simulink model "prius_nocontrol"  (Simulink 6.0)
settings: Solver=ode4  SolverMode=SingleTasking  StartTime=0.0  StopTime=time_final  FixedStep=time_step  RelTol=1e-3  AbsTol=1e-6
values from neighbouring files (symbols this model uses):
  A_frontal = 2.52    [prius_sim_data.m]
  C_d = 0.3    [prius_sim_data.m]
  enable_stop = 1    [prius_sim_data.m]
  eng_consum_fuel = [0 0.654 0.328 0.238 0.232 0.257 0.29 0.323 0.353 0.381 0.407 0.435 0.465 0.501 0.545 0.599 0.665 0.746 0.842 0.957 ... (first row only)    [prius_sim_data.m]
  ess_cap_scale = 1    [prius_sim_data.m]
  ess_fixtemp = 40    [prius_sim_data.m]
  ess_init_soc = soc_init_index(simrun)    [prius_sim_init.m]
  ess_max_ah_cap = [6.0 6.0]    [prius_sim_data.m]
  ess_max_volts = 9    [prius_sim_data.m]
  ess_min_volts = 6    [prius_sim_data.m]
  ess_module_num = 40    [prius_sim_data.m]
  ess_res_scale_coef = [1 0 1 0]    [prius_sim_data.m]
  ess_res_scale_fun = inline('(x(1)*ess_module_num+x(2))/(x(3)*ess_cap_scale+x(4))','x','ess_module_num','ess_cap_scale')    [prius_sim_data.m]
  ess_tmp = [0 25]    [prius_sim_data.m]
  f_rolling = 0.015    [prius_sim_data.m]
  FR = 3.905    [prius_sim_data.m]
  g_eff_map = 0.95*[ 0.88	0.89	0.90	0.91	0.90	0.79	0.79	0.79	0.90	0.91	0.90	0.89	0.88 ... (first row only)    [prius_sim_data.m]
  g_gravity = 9.81    [prius_sim_data.m]
  g_max_spd = [-200000 -10000 -8000 -6500 -5500 -4000 -3500 -3000 -2500 -2000 -1500 -1000 -500 0 500 1000 1500 2000 2500 3000 3500 4000 5500 6500 8000 10000 200000]*(2*pi)/60    [prius_sim_data.m]
  g_max_trq = 1.2*[0.01 14.3 18 22 26 36 41 48 55 55 55 55 55 55 55 55 55 55 55 48 41 36 26 22 18 14.3 0.01]    [prius_sim_data.m]
  gear_no = 4    [prius_sim_data.m]
  m_eff_map = 0.95*[ .905    .905    .905    .905    .905    .905    .905    .905    .905    .905    .905    .905	.905    .905    .905    .905    .905    .905    .905    .905    .905    .905    .905 ... (first row only)    [prius_sim_data.m]
  m_map_spd = [0 500 1000 1500 2000 2500 3000 3500 4000 4500  6000]*(2*pi)/60    [prius_sim_data.m]
  m_max_trq = interp1(m_spd_data,m_max_trq_data,m_map_spd,'linear')    [prius_sim_data.m]
  m_min_volts = 60    [prius_sim_data.m]
  M_total = 1.254*10^3    (= 1254)    [prius_sim_data.m]
  R_tire = 0.287    [prius_sim_data.m]
  rho_air = 1.2    [prius_sim_data.m]
  T2W = inv(W2T)    [prius_sim_data.m]
  time_final = 1*length(cyc_mph(:,2))    [prius_sim_init.m]
  tx_pg_r = 78    [prius_sim_data.m]
  tx_pg_s = 30    [prius_sim_data.m]
undefined symbols (not defined in the file or in its folder): eng_map_trq
settings Model: LastModifiedBy=cpdguest  ExtModeTrigMode=oneshot  ExtModeArmWhenConnect=off  BufferReuse=off
settings SolverCC: InitialStep=0.001
settings DataIOCC: LimitDataPoints=off  SaveOutput=off  SaveTime=off  SignalLoggingName=sigsOut
settings OptimizationCC: BooleanDataType=off  InlineInvariantSignals=off  OptimizeBlockIOStorage=off  BufferReuse=off  ExpressionFolding=off  LocalBlockOutputs=off
settings DebuggingCC: SolverPrmCheckMsg=none
settings HardwareCC: TargetUnknown=on

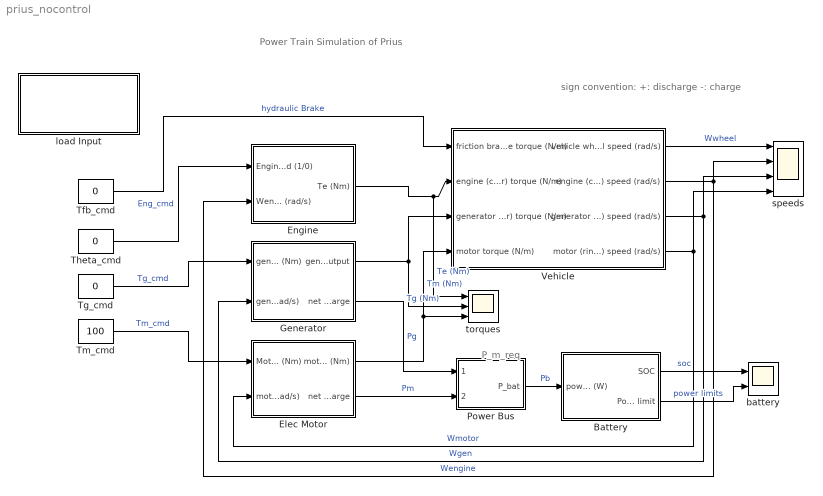
== system prius_nocontrol ==
  note: Power Train Simulation of Prius
  note: P_m_req
  note: sign convention:
      | +: discharge     -: charge
  Battery : Subsystem
      mask Display: disp('Battery')
  Elec Motor : Subsystem
      mask Display: disp('Electric\nMotor')
  Engine : Subsystem
      mask Display: disp('Engine')
  Generator : Subsystem
      mask Display: disp('Generator')
  Power Bus : Subsystem
      mask Display: disp('Power\nBus')
  Tfb_cmd : Constant  Value=0
  Tg_cmd : Constant  Value=0
  Theta_cmd : Constant  Value=0
  Tm_cmd : Constant  Value=100
  Vehicle : Subsystem
      mask Display: disp('Planetary Gear Set\n&\nVehicle')
  battery : Scope  NumInputPorts=2
      settings: TickLabels=on  TimeRange=30  YMin=0~-100  YMax=100~150  SaveName=ScopeData3
  load Input : Subsystem
      settings: OpenFcn=prius_sim_init
      mask Help: This block runs/ndes_init.m file in the main directory
      mask Display: disp('Load Input Data')
  speeds : Scope  NumInputPorts=4
      settings: TickLabels=on  TimeRange=30  YMin=0~-100~-100~-5  YMax=100~150~400~5
  torques : Scope  NumInputPorts=3
      settings: TickLabels=on  TimeRange=30  YMin=0~-100~-100  YMax=100~150~400  SaveName=ScopeData7
  wires:
  Power Bus/1(P_bat) -> Battery/1(power req'd into bus (W))  "Pb"
  Theta_cmd/1 -> Engine/1(Engine on/off cmd (1/0))  "Eng_cmd"
  Tg_cmd/1 -> Generator/1(generator command Torque (Nm))  "Tg_cmd"
  Tm_cmd/1 -> Elec Motor/1(Motor demand Torque (Nm))  "Tm_cmd"
  Elec Motor/2(net Power >0 discharge  <0 charge) -> Power Bus/2(P_motor)  "Pm"
  Generator/2(net Power <0 discharge  >0 charge) -> Power Bus/1(P_generator)  "Pg"
  Tfb_cmd/1 -> Vehicle/1(friction brake torque (N/m))  "hydraulic Brake"
  Engine/1(Te (Nm)) -> Vehicle/2(engine (carrier) torque (N/m)), torques/1  "Te (Nm)"
  Vehicle/2(engine (carrier) speed (rad/s)) -> Engine/2(Wengine (rad/s)), speeds/2  "Wengine"
  Vehicle/3(generator (sun gear) speed (rad/s)) -> Generator/2(generator speed (rad/s)), speeds/3  "Wgen"
  Vehicle/4(motor (ring gear) speed (rad/s)) -> Elec Motor/2(motor speed (rad/s)), speeds/4  "Wmotor"
  Generator/1(generator torque output) -> Vehicle/3(generator (sun gear) torque (N/m)), torques/2  "Tg (Nm)"
  Elec Motor/1(motor torque output (Nm)) -> Vehicle/4(motor torque (N/m)), torques/3  "Tm (Nm)"
  Vehicle/1(vehicle wheel speed (rad/s)) -> speeds/1  "Wwheel"
  Battery/1(SOC) -> battery/1  "soc"
  Battery/2(Power limit) -> battery/2  "power limits"

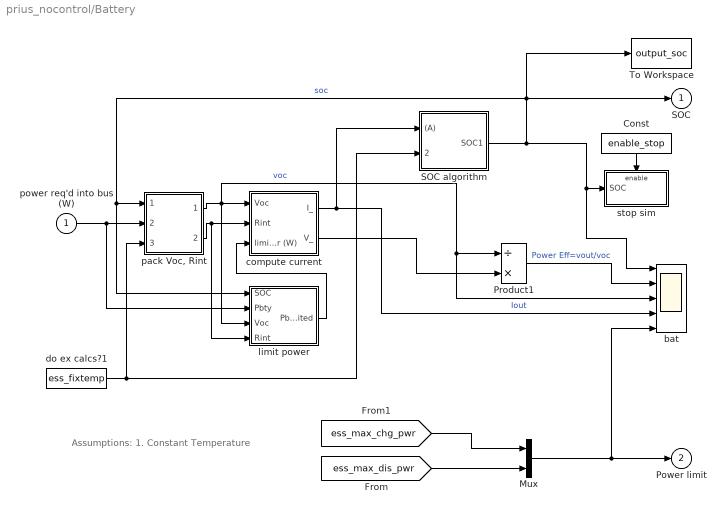
== system prius_nocontrol/Battery ==
  note: Assumptions:
      | 1. Constant Temperature
  power req'd into bus (W) : Inport  Port=1  LatchInput=off
  Const : Constant  Orientation=down  Value=enable_stop
  Mux : Mux  Inputs=2
  Product1 : Product  Inputs=/*  SaturateOnIntegerOverflow=on  InputSameDT=on
  SOC algorithm : Subsystem  AncestorBlock=|
      | lib_energy_storage/Ess Choices/energy
      | storage <ess>/SOC
      | algorithm
      mask Display: disp('SOC\nalgorithm')
  To Workspace : ToWorkspace  VariableName=output_soc  SampleTime=-1  SaveFormat=Array
  bat : Scope  NumInputPorts=5
      settings: TimeRange=367  YMin=0.25~0.75~302~-75~-30000  YMax=0.65~1.2~310~75~25000
  compute current : Subsystem  AncestorBlock=|
      | lib_energy_storage/Ess Choices/energy
      | storage <ess>/compute
      | current
      mask Display: disp('Compute\nCurrent')
  do ex calcs?1 : Constant  Value=ess_fixtemp
  limit power : Subsystem  AncestorBlock=lib_energy_storage/Ess Choices/energy storage <ess>/limit power
      mask Display: disp('Limit\nPower')
  "pack Voc, Rint" : Subsystem  AncestorBlock=|
      | lib_energy_storage/Ess Choices/energy
      | storage <ess>/pack
      | Voc, Rint
      mask Display: disp('Pack\nVoc,Rint')
  stop sim : Subsystem  AncestorBlock=lib_energy_storage/Ess Choices/energy storage <ess>/stop sim  TreatAsAtomicUnit=on
  SOC : Outport  InitialOutput=0
  Power limit : Outport  Port=2  InitialOutput=0
  wires:
  limit power/1("Pbty, limited") -> compute current/3(limited output power (W))
  "pack Voc, Rint"/1(pack open- circuit voltage) -> limit power/3(Voc), compute current/1(Voc), Product1/1, bat/3  "voc"
  "pack Voc, Rint"/2(pack resistance) -> compute current/2(Rint), limit power/4(Rint)
  Const/1 -> stop sim/Enable
  SOC algorithm/1(SOC1) -> limit power/1(SOC), "pack Voc, Rint"/1(SOC (prev)), SOC/1, To Workspace/1, bat/1, stop sim/1(SOC)  "soc"
  compute current/1(I_) -> SOC algorithm/1((A)), bat/4  "Iout"
  power req'd into bus (W)/1 -> "pack Voc, Rint"/2(req'd battery power (W)), limit power/2(Pbty)
  compute current/2(V_) -> Product1/2
  do ex calcs?1/1 -> "pack Voc, Rint"/3(mod tmp   (C)), SOC algorithm/2(tmp (C))
  Mux/1 -> Power limit/1, bat/5
  Product1/1 -> bat/2  "Power Eff=vout/voc"
  [ess_max_dis_pwr] -> Mux/2
  [ess_max_chg_pwr] -> Mux/1

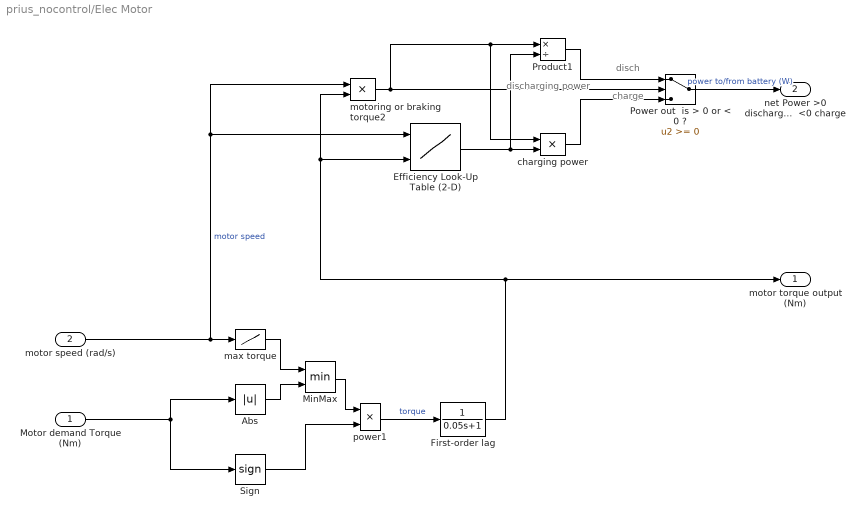
== system prius_nocontrol/Elec Motor ==
  note: disch
  note: charge
  note: discharging
      | power
  Motor demand Torque (Nm) : Inport  Port=1  LatchInput=off
  motor speed (rad/s) : Inport  Port=2  LatchInput=off
  Abs : Abs  SaturateOnIntegerOverflow=on
  Efficiency Look-Up Table (2-D) : Lookup2D  DialogController=Simulink.DDGSource  RowIndex=m_map_spd  ColumnIndex=m_map_trq  OutputValues=m_eff_map  SaturateOnIntegerOverflow=on  InputSameDT=on
  First-order lag : TransferFcn  Denominator=[0.05 1]
  MinMax : MinMax  Inputs=2  SaturateOnIntegerOverflow=on  InputSameDT=on
  Power out  is > 0 or < 0 ? : Switch  SaturateOnIntegerOverflow=on  InputSameDT=on
  Product1 : Product  Inputs=*/  SaturateOnIntegerOverflow=on  InputSameDT=on
  Sign : Signum
  charging power : Product  SaturateOnIntegerOverflow=on  InputSameDT=on
  max torque : Lookup  DialogController=Simulink.DDGSource  InputValues=m_map_spd  OutputValues=m_max_trq  SaturateOnIntegerOverflow=on
  motoring or braking torque2 : Product  SaturateOnIntegerOverflow=on  InputSameDT=on
  power1 : Product  SaturateOnIntegerOverflow=on  InputSameDT=on
  motor torque output (Nm) : Outport  InitialOutput=0
  net Power >0 discharge  <0 charge : Outport  Port=2  InitialOutput=0
  wires:
  charging power/1 -> Power out  is > 0 or < 0 ?/3
  Product1/1 -> Power out  is > 0 or < 0 ?/1
  Power out  is > 0 or < 0 ?/1 -> net Power >0 discharge  <0 charge/1  "power to/from battery (W)"
  motor speed (rad/s)/1 -> Efficiency Look-Up Table (2-D)/1, motoring or braking torque2/1, max torque/1  "motor speed"
  Motor demand Torque (Nm)/1 -> Abs/1, Sign/1
  power1/1 -> First-order lag/1  "torque"
  Efficiency Look-Up Table (2-D)/1 -> Product1/2, charging power/2
  motoring or braking torque2/1 -> Product1/1, charging power/1, Power out  is > 0 or < 0 ?/2
  Abs/1 -> MinMax/2
  max torque/1 -> MinMax/1
  MinMax/1 -> power1/1
  Sign/1 -> power1/2
  First-order lag/1 -> Efficiency Look-Up Table (2-D)/2, motoring or braking torque2/2, motor torque output (Nm)/1

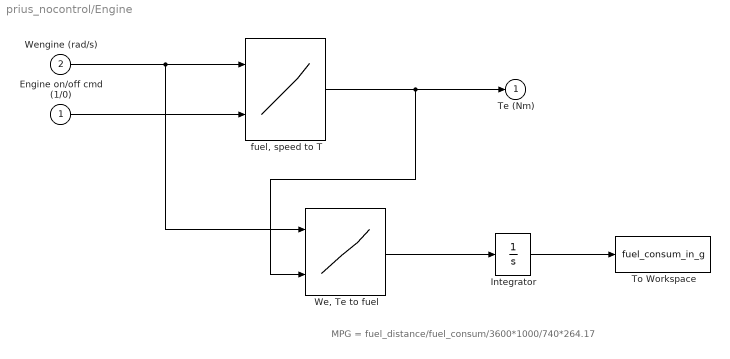
== system prius_nocontrol/Engine ==
  note: MPG = fuel_distance/fuel_consum/3600*1000/740*264.17
  Engine on/off cmd (1/0) : Inport  Port=1  LatchInput=off
  Wengine (rad/s) : Inport  Port=2  LatchInput=off
  Integrator : Integrator  UpperSaturationLimit=20.5  LowerSaturationLimit=0
  To Workspace : ToWorkspace  VariableName=fuel_consum_in_g  SampleTime=time_final  SaveFormat=Array
  "We, Te to fuel" : Lookup2D  DialogController=Simulink.DDGSource  RowIndex=eng_consum_spd  ColumnIndex=eng_consum_trq  OutputValues=eng_consum_fuel  SaturateOnIntegerOverflow=on  InputSameDT=on
  "fuel, speed to T" : Lookup2D  DialogController=Simulink.DDGSource  RowIndex=eng_map_spd  ColumnIndex=eng_map_fuel  OutputValues=eng_map_trq  SaturateOnIntegerOverflow=on  InputSameDT=on
  Te (Nm) : Outport
  wires:
  Engine on/off cmd (1/0)/1 -> "fuel, speed to T"/2
  Wengine (rad/s)/1 -> "fuel, speed to T"/1, "We, Te to fuel"/1
  "fuel, speed to T"/1 -> Te (Nm)/1, "We, Te to fuel"/2
  "We, Te to fuel"/1 -> Integrator/1
  Integrator/1 -> To Workspace/1

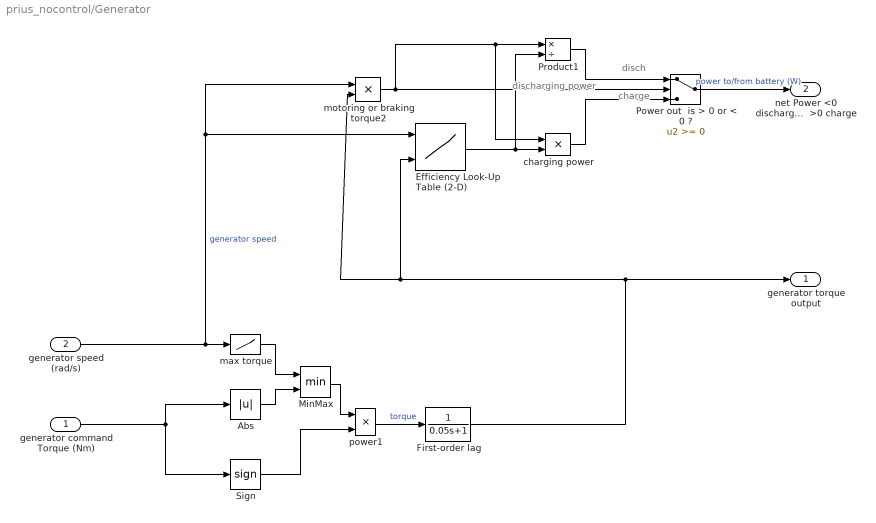
== system prius_nocontrol/Generator ==
  note: disch
  note: charge
  note: discharging
      | power
  generator command Torque (Nm) : Inport  Port=1  LatchInput=off
  generator speed (rad/s) : Inport  Port=2  LatchInput=off
  Abs : Abs  SaturateOnIntegerOverflow=on
  Efficiency Look-Up Table (2-D) : Lookup2D  DialogController=Simulink.DDGSource  RowIndex=g_map_spd  ColumnIndex=g_map_trq  OutputValues=g_eff_map  SaturateOnIntegerOverflow=on  InputSameDT=on
  First-order lag : TransferFcn  Denominator=[0.05 1]
  MinMax : MinMax  Inputs=2  SaturateOnIntegerOverflow=on  InputSameDT=on
  Power out  is > 0 or < 0 ? : Switch  SaturateOnIntegerOverflow=on  InputSameDT=on
  Product1 : Product  Inputs=*/  SaturateOnIntegerOverflow=on  InputSameDT=on
  Sign : Signum
  charging power : Product  SaturateOnIntegerOverflow=on  InputSameDT=on
  max torque : Lookup  DialogController=Simulink.DDGSource  InputValues=g_max_spd  OutputValues=g_max_trq  SaturateOnIntegerOverflow=on
  motoring or braking torque2 : Product  SaturateOnIntegerOverflow=on  InputSameDT=on
  power1 : Product  SaturateOnIntegerOverflow=on  InputSameDT=on
  generator torque output : Outport  InitialOutput=0
  net Power <0 discharge  >0 charge : Outport  Port=2  InitialOutput=0
  wires:
  charging power/1 -> Power out  is > 0 or < 0 ?/3
  Product1/1 -> Power out  is > 0 or < 0 ?/1
  Power out  is > 0 or < 0 ?/1 -> net Power <0 discharge  >0 charge/1  "power to/from battery (W)"
  generator speed (rad/s)/1 -> Efficiency Look-Up Table (2-D)/1, motoring or braking torque2/1, max torque/1  "generator speed"
  generator command Torque (Nm)/1 -> Abs/1, Sign/1
  power1/1 -> First-order lag/1  "torque"
  Efficiency Look-Up Table (2-D)/1 -> Product1/2, charging power/2
  motoring or braking torque2/1 -> Product1/1, charging power/1, Power out  is > 0 or < 0 ?/2
  Abs/1 -> MinMax/2
  max torque/1 -> MinMax/1
  MinMax/1 -> power1/1
  Sign/1 -> power1/2
  First-order lag/1 -> generator torque output/1, Efficiency Look-Up Table (2-D)/2, motoring or braking torque2/2

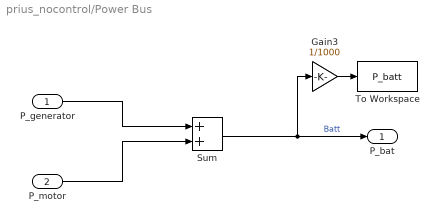
== system prius_nocontrol/Power Bus ==
  P_generator : Inport  Port=1  LatchInput=off
  P_motor : Inport  Port=2  LatchInput=off
  Gain3 : Gain  Gain=1/1000  SaturateOnIntegerOverflow=on
  Sum : Sum  SaturateOnIntegerOverflow=on  InputSameDT=on
  To Workspace : ToWorkspace  VariableName=P_batt  SampleTime=-1  SaveFormat=Array
  P_bat : Outport  InitialOutput=0
  wires:
  P_generator/1 -> Sum/1
  P_motor/1 -> Sum/2
  Sum/1 -> P_bat/1, Gain3/1  "Batt"
  Gain3/1 -> To Workspace/1

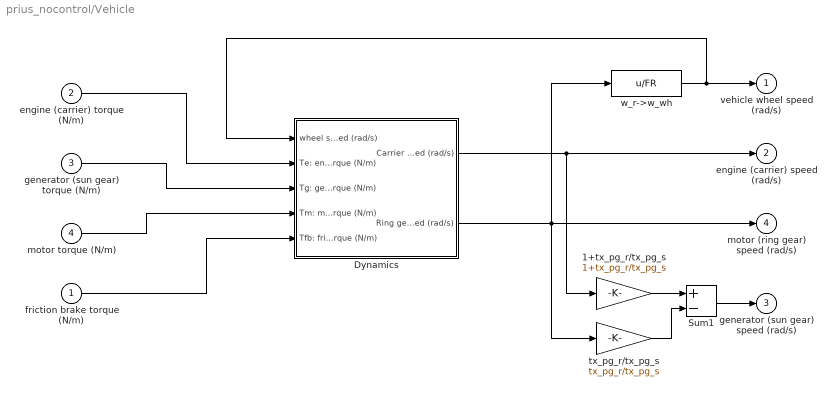
== system prius_nocontrol/Vehicle ==
  friction brake torque (N/m) : Inport  Port=1  LatchInput=off
  engine (carrier) torque (N/m) : Inport  Port=2  LatchInput=off
  generator (sun gear) torque (N/m) : Inport  Port=3  LatchInput=off
  motor torque (N/m) : Inport  Port=4  LatchInput=off
  1+tx_pg_r/tx_pg_s : Gain  Gain=1+tx_pg_r/tx_pg_s  SaturateOnIntegerOverflow=on
  Dynamics : Subsystem
      mask Display: disp('Dynamic Model\nTwo DOF')
  Sum1 : Sum  Inputs=+-  SaturateOnIntegerOverflow=on  InputSameDT=on
  tx_pg_r/tx_pg_s : Gain  Gain=tx_pg_r/tx_pg_s  SaturateOnIntegerOverflow=on
  w_r->w_wh : Fcn  Expr=u/FR
  vehicle wheel speed (rad/s) : Outport
  engine (carrier) speed (rad/s) : Outport  Port=2
  generator (sun gear) speed (rad/s) : Outport  Port=3
  motor (ring gear) speed (rad/s) : Outport  Port=4
  wires:
  tx_pg_r/tx_pg_s/1 -> Sum1/2
  1+tx_pg_r/tx_pg_s/1 -> Sum1/1
  engine (carrier) torque (N/m)/1 -> Dynamics/2(Te: engine (carrier) torque (N/m))
  motor torque (N/m)/1 -> Dynamics/4(Tm: motor torque (N/m))
  friction brake torque (N/m)/1 -> Dynamics/5("Tfb: friction brake torque (N/m) ")
  w_r->w_wh/1 -> vehicle wheel speed (rad/s)/1, Dynamics/1(wheel speed (rad/s))
  generator (sun gear) torque (N/m)/1 -> Dynamics/3(Tg: generator (sun gear) torque (N/m))
  Sum1/1 -> generator (sun gear) speed (rad/s)/1
  Dynamics/1(Carrier speed (rad/s)) -> engine (carrier) speed (rad/s)/1, 1+tx_pg_r/tx_pg_s/1
  Dynamics/2(Ring gear speed (rad/s)) -> w_r->w_wh/1, motor (ring gear) speed (rad/s)/1, tx_pg_r/tx_pg_s/1

== system prius_nocontrol/load Input ==
  note: double_click to load

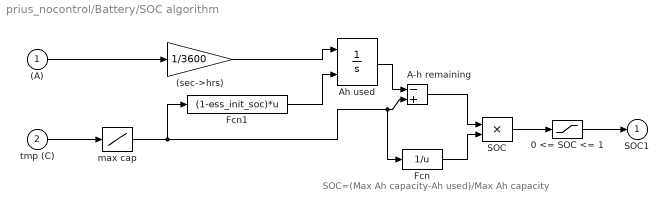
== system prius_nocontrol/Battery/SOC algorithm ==
  note: SOC=(Max Ah capacity-Ah used)/Max Ah capacity
  (A) : Inport  Port=1  LatchInput=off
  tmp (C) : Inport  Port=2  LatchInput=off
  (sec->hrs) : Gain  Gain=1/3600  SaturateOnIntegerOverflow=on
  0 <= SOC <= 1 : Saturate  UpperLimit=1  LowerLimit=0
  A-h remaining : Sum  Inputs=-+  SaturateOnIntegerOverflow=on  InputSameDT=on
  Ah used : Integrator  InitialConditionSource=external  InitialCondition=(1-ess_init_soc)*ess_max_ah_cap
  Fcn : Fcn  Expr=1/u
  Fcn1 : Fcn  Expr=(1-ess_init_soc)*u
  SOC : Product  SaturateOnIntegerOverflow=on  InputSameDT=on
  max cap : Lookup  DialogController=Simulink.DDGSource  InputValues=ess_tmp  OutputValues=ess_max_ah_cap*ess_cap_scale  SaturateOnIntegerOverflow=on
  SOC1 : Outport  InitialOutput=0
  wires:
  (A)/1 -> (sec->hrs)/1
  (sec->hrs)/1 -> Ah used/1
  Ah used/1 -> A-h remaining/1
  Fcn/1 -> SOC/2
  SOC/1 -> 0 <= SOC <= 1/1
  A-h remaining/1 -> SOC/1
  0 <= SOC <= 1/1 -> SOC1/1
  tmp (C)/1 -> max cap/1
  max cap/1 -> A-h remaining/2, Fcn/1, Fcn1/1
  Fcn1/1 -> Ah used/2

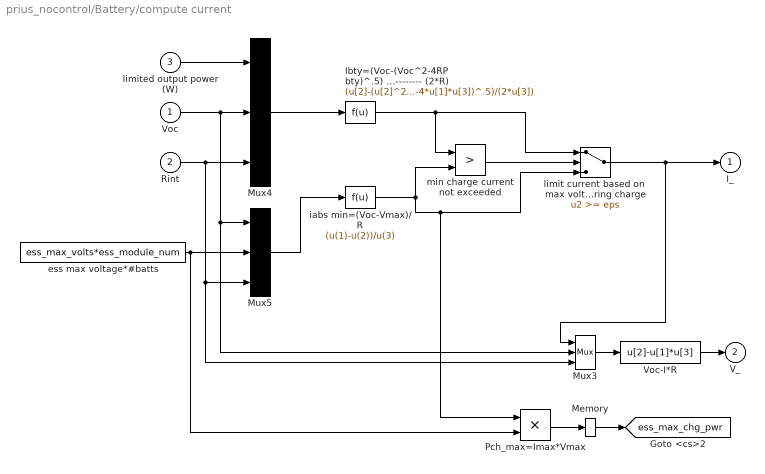
== system prius_nocontrol/Battery/compute current ==
  Voc : Inport  Port=1  LatchInput=off
  Rint : Inport  Port=2  LatchInput=off
  limited output power (W) : Inport  Port=3  LatchInput=off
  Ibty=(Voc-(Voc^2-4RPbty)^.5)        ----------------------------- (2*R) : Fcn  Expr=(u[2]-(u[2]^2-4*u[1]*u[3])^.5)/(2*u[3])
  Memory : Memory
  Mux3 : Mux  Inputs=3
  Mux4 : Mux  Inputs=3
  Mux5 : Mux  Inputs=3
  Pch_max=Imax*Vmax : Product  SaturateOnIntegerOverflow=on  InputSameDT=on
  Voc-I*R : Fcn  Expr=u[2]-u[1]*u[3]
  ess max voltage*#batts : Constant  Value=ess_max_volts*ess_module_num
  iabs min=(Voc-Vmax)/R : Fcn  Expr=(u(1)-u(2))/u(3)
  limit current based on  max voltage during charge : Switch  Threshold=eps  SaturateOnIntegerOverflow=on  InputSameDT=on
  min charge current not exceeded : RelationalOperator  Operator=>  InputSameDT=on
  I_ : Outport  InitialOutput=0
  V_ : Outport  Port=2  InitialOutput=0
  tag scope: ess_max_chg_pwr=global
  wires:
  limited output power (W)/1 -> Mux4/1
  Voc/1 -> Mux4/2, Mux3/2, Mux5/1
  Rint/1 -> Mux4/3, Mux3/3, Mux5/3
  Ibty=(Voc-(Voc^2-4RPbty)^.5)        ----------------------------- (2*R)/1 -> min charge current not exceeded/1, limit current based on  max voltage during charge/1
  iabs min=(Voc-Vmax)/R/1 -> min charge current not exceeded/2, limit current based on  max voltage during charge/3, Pch_max=Imax*Vmax/1
  limit current based on  max voltage during charge/1 -> Mux3/1, I_/1
  min charge current not exceeded/1 -> limit current based on  max voltage during charge/2
  Mux3/1 -> Voc-I*R/1
  Voc-I*R/1 -> V_/1
  Mux4/1 -> Ibty=(Voc-(Voc^2-4RPbty)^.5)        ----------------------------- (2*R)/1
  Mux5/1 -> iabs min=(Voc-Vmax)/R/1
  ess max voltage*#batts/1 -> Mux5/2, Pch_max=Imax*Vmax/2
  Pch_max=Imax*Vmax/1 -> Memory/1
  Memory/1 -> [ess_max_chg_pwr]

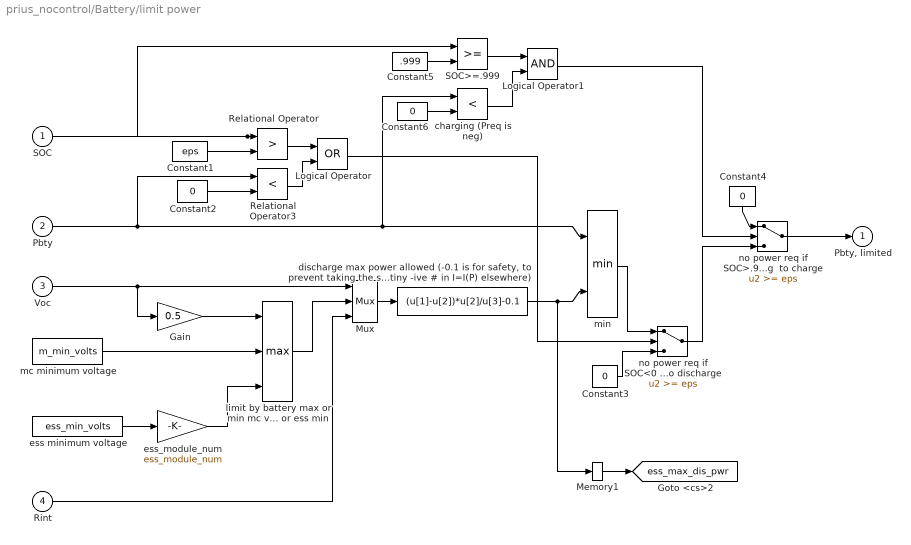
== system prius_nocontrol/Battery/limit power ==
  SOC : Inport  Port=1  LatchInput=off
  Pbty : Inport  Port=2  LatchInput=off
  Voc : Inport  Port=3  LatchInput=off
  Rint : Inport  Port=4  LatchInput=off
  Constant1 : Constant  Value=eps
  Constant2 : Constant  Value=0
  Constant3 : Constant  Value=0
  Constant4 : Constant  Orientation=down  Value=0
  Constant5 : Constant  Value=.999
  Constant6 : Constant  Value=0
  Gain : Gain  Gain=0.5  SaturateOnIntegerOverflow=on
  Logical Operator : Logic  Operator=OR
  Logical Operator1 : Logic
  Memory1 : Memory
  Mux : Mux  Inputs=3
  Relational Operator : RelationalOperator  Operator=>  InputSameDT=on
  Relational Operator3 : RelationalOperator  Operator=<  InputSameDT=on
  SOC>=.999 : RelationalOperator  InputSameDT=on
  charging (Preq is neg) : RelationalOperator  Operator=<  InputSameDT=on
  "discharge max power allowed (-0.1 is for safety, to prevent taking the square of a tiny -ive # in I=I(P) elsewhere)" : Fcn  Expr=(u[1]-u[2])*u[2]/u[3]-0.1
  ess minimum voltage : Constant  Value=ess_min_volts
  ess_module_num : Gain  Gain=ess_module_num  SaturateOnIntegerOverflow=on
  limit by battery max or min mc voltage or ess min : MinMax  Function=max  Inputs=3  SaturateOnIntegerOverflow=on  InputSameDT=on
  mc minimum voltage : Constant  Value=m_min_volts
  min : MinMax  Inputs=2  SaturateOnIntegerOverflow=on  InputSameDT=on
  no power req if SOC<0 and trying  to discharge : Switch  Threshold=eps  SaturateOnIntegerOverflow=on  InputSameDT=on
  no power req if SOC>.999 and trying  to charge : Switch  Threshold=eps  SaturateOnIntegerOverflow=on  InputSameDT=on
  "Pbty, limited" : Outport  InitialOutput=0
  tag scope: ess_max_dis_pwr=global
  wires:
  Constant1/1 -> Relational Operator/2
  Relational Operator/1 -> Logical Operator/1
  Pbty/1 -> Relational Operator3/1, charging (Preq is neg)/1, min/1
  Constant2/1 -> Relational Operator3/2
  Relational Operator3/1 -> Logical Operator/2
  Constant3/1 -> no power req if SOC<0 and trying  to discharge/3
  Logical Operator/1 -> no power req if SOC<0 and trying  to discharge/2
  Voc/1 -> Mux/1, Gain/1
  min/1 -> no power req if SOC<0 and trying  to discharge/1
  Mux/1 -> "discharge max power allowed (-0.1 is for safety, to prevent taking the square of a tiny -ive # in I=I(P) elsewhere)"/1
  limit by battery max or min mc voltage or ess min/1 -> Mux/2
  "discharge max power allowed (-0.1 is for safety, to prevent taking the square of a tiny -ive # in I=I(P) elsewhere)"/1 -> min/2, Memory1/1
  mc minimum voltage/1 -> limit by battery max or min mc voltage or ess min/2
  Rint/1 -> Mux/3
  Gain/1 -> limit by battery max or min mc voltage or ess min/1
  ess minimum voltage/1 -> ess_module_num/1
  ess_module_num/1 -> limit by battery max or min mc voltage or ess min/3
  SOC/1 -> Relational Operator/1, SOC>=.999/1
  SOC>=.999/1 -> Logical Operator1/1
  Constant6/1 -> charging (Preq is neg)/2
  charging (Preq is neg)/1 -> Logical Operator1/2
  Constant5/1 -> SOC>=.999/2
  Constant4/1 -> no power req if SOC>.999 and trying  to charge/1
  no power req if SOC<0 and trying  to discharge/1 -> no power req if SOC>.999 and trying  to charge/3
  no power req if SOC>.999 and trying  to charge/1 -> "Pbty, limited"/1
  Logical Operator1/1 -> no power req if SOC>.999 and trying  to charge/2
  Memory1/1 -> [ess_max_dis_pwr]

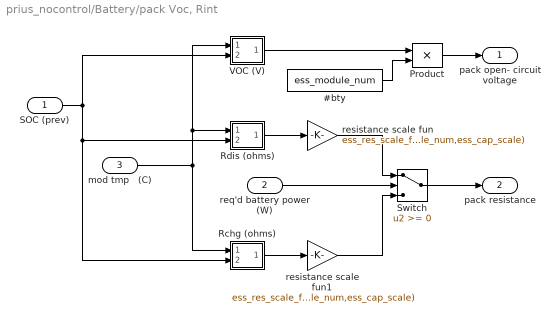
== system prius_nocontrol/Battery/pack Voc, Rint ==
  SOC (prev) : Inport  Port=1  LatchInput=off
  req'd battery power (W) : Inport  Port=2  LatchInput=off
  mod tmp   (C) : Inport  Port=3  LatchInput=off
  #bty : Constant  Value=ess_module_num
  Product : Product  SaturateOnIntegerOverflow=on  InputSameDT=on
  Rchg (ohms) : Subsystem  mask(2-D Table Lookup){@1=ess_tmp, @2=ess_soc, @3=ess_r_chg}
      mask prompts: @1 "X Index"; @2 "Y Index"; @3 "Table"
      mask help:
      | Two Dimensional Table Lookup
      | The first input corresponds to X Index and the second input corresponds to the Y Index
      mask init:
      | xindex=@1; yindex=@2; table=@3; sftab2chk(xindex,yindex,table);
      mask Help: This block returns a linearly interpolated intersection from the table using the X index (which corresponds to the rows of the table) and the Y index (which corresponds to the columns of the table).  Extrapolation is used.
      mask Display: plot(-10,-10,110,110,[90,50,10],[90,40,30],[90,50,10],[50,26,20],[90,50,10],[22,13,10])
  Rdis (ohms) : Subsystem  mask(2-D Table Lookup){@1=ess_tmp, @2=ess_soc, @3=ess_r_dis}
      mask prompts: @1 "X Index"; @2 "Y Index"; @3 "Table"
      mask help:
      | Two Dimensional Table Lookup
      | The first input corresponds to X Index and the second input corresponds to the Y Index
      mask init:
      | xindex=@1; yindex=@2; table=@3; sftab2chk(xindex,yindex,table);
      mask Help: This block returns a linearly interpolated intersection from the table using the X index (which corresponds to the rows of the table) and the Y index (which corresponds to the columns of the table).  Extrapolation is used.
      mask Display: plot(-10,-10,110,110,[90,50,10],[90,40,30],[90,50,10],[50,26,20],[90,50,10],[22,13,10])
  Switch : Switch  SaturateOnIntegerOverflow=on  InputSameDT=on
  VOC (V) : Subsystem  mask(2-D Table Lookup){@1=ess_tmp, @2=ess_soc, @3=ess_voc}
      mask prompts: @1 "X Index"; @2 "Y Index"; @3 "Table"
      mask help:
      | Two Dimensional Table Lookup
      | The first input corresponds to X Index and the second input corresponds to the Y Index
      mask init:
      | xindex=@1; yindex=@2; table=@3; sftab2chk(xindex,yindex,table);
      mask Help: This block returns a linearly interpolated intersection from the table using the X index (which corresponds to the rows of the table) and the Y index (which corresponds to the columns of the table).  Extrapolation is used.
      mask Display: plot(-10,-10,110,110,[90,50,10],[90,40,30],[90,50,10],[50,26,20],[90,50,10],[22,13,10])
  resistance scale fun : Gain  Gain=ess_res_scale_fun(ess_res_scale_coef,ess_module_num,ess_cap_scale)  SaturateOnIntegerOverflow=on
  resistance scale fun1 : Gain  Gain=ess_res_scale_fun(ess_res_scale_coef,ess_module_num,ess_cap_scale)  SaturateOnIntegerOverflow=on
  pack open- circuit voltage : Outport  InitialOutput=0
  pack resistance : Outport  Port=2  InitialOutput=0
  wires:
  resistance scale fun1/1 -> Switch/3
  Rchg (ohms)/1(table out) -> resistance scale fun1/1
  resistance scale fun/1 -> Switch/1
  Rdis (ohms)/1(table out) -> resistance scale fun/1
  Switch/1 -> pack resistance/1
  #bty/1 -> Product/2
  Product/1 -> pack open- circuit voltage/1
  VOC (V)/1(table out) -> Product/1
  req'd battery power (W)/1 -> Switch/2
  SOC (prev)/1 -> VOC (V)/2(y0), Rdis (ohms)/2(y0), Rchg (ohms)/2(y0)
  mod tmp   (C)/1 -> VOC (V)/1(x0), Rdis (ohms)/1(x0), Rchg (ohms)/1(x0)

== system prius_nocontrol/Battery/stop sim ==
  SOC : Inport  Port=1  LatchInput=off
  Enable : EnablePort
  Const : Constant  Orientation=up  Value=.001
  Relational Operator : RelationalOperator  Operator=<  InputSameDT=on
  Stop Simulation : Stop
  wires:
  Const/1 -> Relational Operator/2
  SOC/1 -> Relational Operator/1
  Relational Operator/1 -> Stop Simulation/1

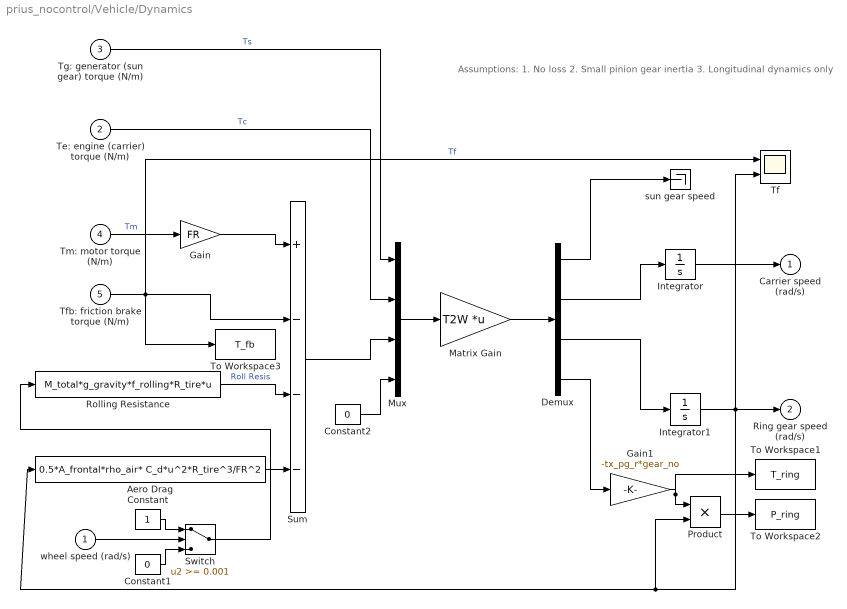
== system prius_nocontrol/Vehicle/Dynamics ==
  note: Assumptions:
      | 1. No loss
      | 2. Small pinion gear inertia
      | 3. Longitudinal dynamics only
  wheel speed (rad/s) : Inport  Port=1  LatchInput=off
  Te: engine (carrier) torque (N/m) : Inport  Port=2  LatchInput=off
  Tg: generator (sun gear) torque (N/m) : Inport  Port=3  LatchInput=off
  Tm: motor torque (N/m) : Inport  Port=4  LatchInput=off
  "Tfb: friction brake torque (N/m) " : Inport  Port=5  LatchInput=off
  Aero Drag : Fcn  Expr=0.5*A_frontal*rho_air* C_d*u^2*R_tire^3/FR^2
  Constant : Constant
  Constant1 : Constant  Value=0
  Constant2 : Constant  Value=0
  Demux : Demux
  Gain : Gain  Gain=FR  SaturateOnIntegerOverflow=on
  Gain1 : Gain  Gain=-tx_pg_r*gear_no  SaturateOnIntegerOverflow=on
  Integrator : Integrator  InitialCondition=1000*2*pi/60  LimitOutput=on  LowerSaturationLimit=0
  Integrator1 : Integrator  LimitOutput=on  LowerSaturationLimit=0
  Matrix Gain : Gain  Gain=T2W  Multiplication=Matrix(K*u)  SaturateOnIntegerOverflow=on
  Mux : Mux
  Product : Product  SaturateOnIntegerOverflow=on  InputSameDT=on
  Rolling Resistance : Fcn  Expr=M_total*g_gravity*f_rolling*R_tire*u
  Sum : Sum  Inputs=+---  SaturateOnIntegerOverflow=on
  Switch : Switch  Threshold=0.001  SaturateOnIntegerOverflow=on
  Tf : Scope  NumInputPorts=2
      settings: TickLabels=on  TimeRange=30  YMin=-20000~-50000  YMax=100000~50000  SaveName=ScopeData2
  To Workspace1 : ToWorkspace  VariableName=T_ring  SampleTime=-1  SaveFormat=Array
  To Workspace2 : ToWorkspace  VariableName=P_ring  SampleTime=-1  SaveFormat=Array
  To Workspace3 : ToWorkspace  VariableName=T_fb  SampleTime=-1  SaveFormat=Array
  sun gear speed : Terminator
  Carrier speed (rad/s) : Outport  InitialOutput=0
  Ring gear speed (rad/s) : Outport  Port=2  InitialOutput=0
  wires:
  Demux/2 -> Integrator/1
  Integrator/1 -> Carrier speed (rad/s)/1
  Demux/3 -> Integrator1/1
  Integrator1/1 -> Ring gear speed (rad/s)/1, Tf/2, Aero Drag/1, Product/2
  Rolling Resistance/1 -> Sum/3  "Roll Resis"
  Aero Drag/1 -> Sum/4
  wheel speed (rad/s)/1 -> Switch/2
  Tm: motor torque (N/m)/1 -> Gain/1  "Tm"
  Constant1/1 -> Switch/3
  Constant/1 -> Switch/1
  Switch/1 -> Rolling Resistance/1
  Gain/1 -> Sum/1
  "Tfb: friction brake torque (N/m) "/1 -> Sum/2, Tf/1, To Workspace3/1  "Tf"
  Mux/1 -> Matrix Gain/1
  Tg: generator (sun gear) torque (N/m)/1 -> Mux/1  "Ts"
  Te: engine (carrier) torque (N/m)/1 -> Mux/2  "Tc"
  Sum/1 -> Mux/3
  Constant2/1 -> Mux/4
  Matrix Gain/1 -> Demux/1
  Demux/1 -> sun gear speed/1
  Demux/4 -> Gain1/1
  Gain1/1 -> To Workspace1/1, Product/1
  Product/1 -> To Workspace2/1

== system prius_nocontrol/Battery/pack Voc, Rint/Rchg (ohms) ==
  x0 : Inport  Port=1  LatchInput=off
  y0 : Inport  Port=2  LatchInput=off
  Mux : Mux  Inputs=2
  S-function : S-Function  FunctionName=sftable2  Parameters=xindex, yindex, table
  table out : Outport  InitialOutput=0
  wires:
  y0/1 -> Mux/2
  S-function/1 -> table out/1
  x0/1 -> Mux/1
  Mux/1 -> S-function/1

== system prius_nocontrol/Battery/pack Voc, Rint/Rdis (ohms) ==
  x0 : Inport  Port=1  LatchInput=off
  y0 : Inport  Port=2  LatchInput=off
  Mux : Mux  Inputs=2
  S-function : S-Function  FunctionName=sftable2  Parameters=xindex, yindex, table
  table out : Outport  InitialOutput=0
  wires:
  y0/1 -> Mux/2
  S-function/1 -> table out/1
  x0/1 -> Mux/1
  Mux/1 -> S-function/1

== system prius_nocontrol/Battery/pack Voc, Rint/VOC (V) ==
  x0 : Inport  Port=1  LatchInput=off
  y0 : Inport  Port=2  LatchInput=off
  Mux : Mux  Inputs=2
  S-function : S-Function  FunctionName=sftable2  Parameters=xindex, yindex, table
  table out : Outport  InitialOutput=0
  wires:
  y0/1 -> Mux/2
  S-function/1 -> table out/1
  x0/1 -> Mux/1
  Mux/1 -> S-function/1
